simulink model "Scatola2"  (R2019a)
settings: Solver=VariableStepAuto  StartTime=0.0  StopTime=10.0  RelTol=1e-3
settings Model: Creator=anton  LastModifiedBy=anton

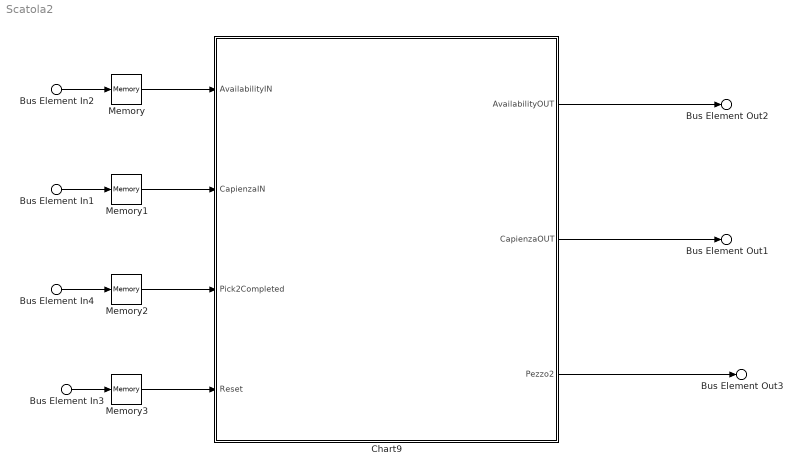
== system Scatola2 ==
  Bus Element In1 : Inport  PortName=CapienzaIN
  Bus Element In3 : Inport  Port=2  PortName=Reset
  Bus Element In4 : Inport  Port=3  PortName=Pick2Completed
  Bus Element In2 : Inport  Port=4  PortName=AvailabilityIN
  Chart9 : Stateflow chart  BlockKeywords=__PRM__SERIALIZED__DATA__:Stateflow Chart,Stateflow Diagram  TreatAsAtomicUnit=on
  Memory{,1..3} (4 alike) : Memory
  Bus Element Out1 : Outport  PortName=Capienza2OUT
  Bus Element Out2 : Outport  Port=2  PortName=AvailabilityOUT
  Bus Element Out3 : Outport  Port=3  PortName=Pezzo
  wires:
  Chart9/2(CapienzaOUT) -> Bus Element Out1/1
  Chart9/1(AvailabilityOUT) -> Bus Element Out2/1
  Chart9/3(Pezzo2) -> Bus Element Out3/1
  Bus Element In2/1 -> Memory/1
  Memory/1 -> Chart9/1(AvailabilityIN)
  Bus Element In1/1 -> Memory1/1
  Memory1/1 -> Chart9/2(CapienzaIN)
  Bus Element In4/1 -> Memory2/1
  Memory2/1 -> Chart9/3(Pick2Completed)
  Bus Element In3/1 -> Memory3/1
  Memory3/1 -> Chart9/4(Reset)

== stateflow chart Scatola2/Chart9 ==
  state Idle
    CapienzaOUT=4;
    AvailabilityOUT=AvailabilityIN;
    pause(0.1);
  state Capienza4
    CapienzaOUT=4;
    Pezzo2=1;
    AvailabilityOUT=AvailabilityIN;
    pause(0.1);
  state Waiting3
  state Capienza3
    CapienzaOUT=3;
    Pezzo2=1;
    AvailabilityOUT=AvailabilityIN;
    pause(0.1);
  state Waiting2
  state Capienza2
    CapienzaOUT=2;
    Pezzo2=1;
    AvailabilityOUT=AvailabilityIN;
    pause(0.1);
  state Waiting
  state Capienza1
    CapienzaOUT=1;
    Pezzo2=1;
    AvailabilityOUT=AvailabilityIN;
    pause(0.1);
  state Waiting1
  state Capienza0
    CapienzaOUT=0;
    Pezzo2=0;
    AvailabilityOUT=AvailabilityIN;
    pause(0.1);
  (default) -> Idle
  Capienza0 -> Idle : [CapienzaIN==1]
  Idle -> Capienza4
  Capienza4 -> Waiting3 : [Pick2Completed==1]
  Waiting3 -> Capienza3 : [Reset==1]
  Capienza3 -> Waiting2 : [Pick2Completed==1]
  Waiting2 -> Capienza2 : [Reset==1]
  Capienza2 -> Waiting : [Pick2Completed==1]
  Waiting -> Capienza1 : [Reset==1]
  Capienza1 -> Waiting1 : [Pick2Completed==1]
  Waiting1 -> Capienza0 : [Reset==1]
  data: AvailabilityIN input; CapienzaIN input; Pick2Completed input; Reset input; AvailabilityOUT output; CapienzaOUT output; Pezzo2 output
